simulink model "CanBusRagnar2020b"  (R2020b)
settings: Solver=VariableStepAuto  StartTime=0.0  StopTime=5.0  RelTol=1e-3
values from neighbouring files (symbols this model uses):
  F_mimo = -place(A,B,Desired_poles)    [SS_MIMO.m]    (also in controller_code.m = [ -230.9401         0         0         0  -34.4133         )
  sys_mimo = ss(A,B,C,0)    [SS_MIMO.m]
libraries: truetime x6, simulink_extras x4, dspsrcs4 x1
settings Model: Creator=mozzr  LastModifiedBy=krist
settings DebuggingCC: SFMachineParentedDataDiag=error

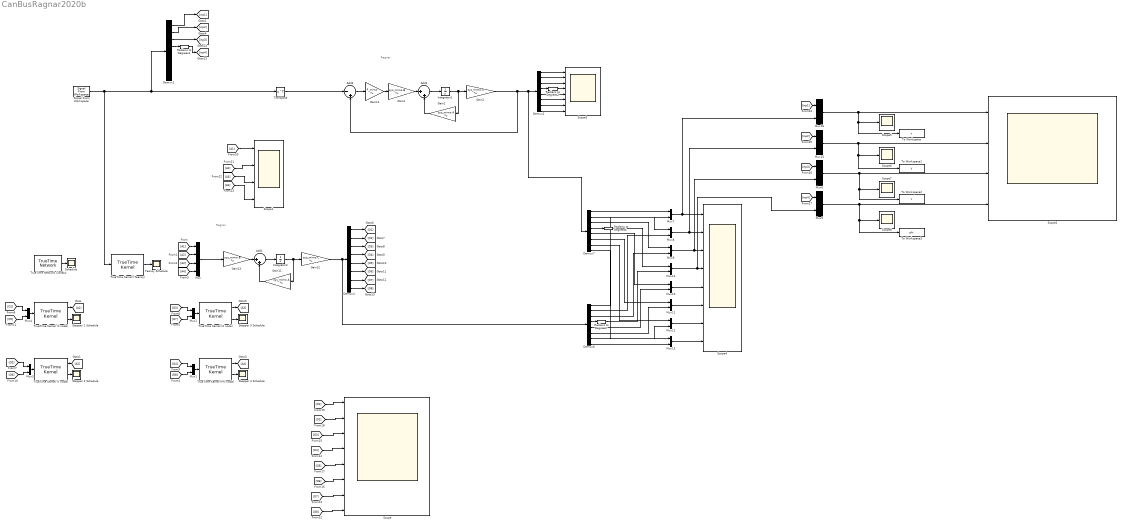
== system CanBusRagnar2020b ==
  note: Ragnar
  note: Ragnar
  Add1 : Sum  Inputs=|++
  Add2 : Sum  Inputs=|++
  Add3 : Sum  Inputs=|-+
  Demux{1..2,4,6..7} (5 alike) : Demux  Outputs=8
  Gain1 : Gain  Gain=sys_mimo.A  Multiplication=Matrix(K*u)
  Gain11 : Gain  Gain=sys_mimo.A  Multiplication=Matrix(K*u)
  Gain12 : Gain  Gain=sys_mimo.C  Multiplication=Matrix(K*u)
  Gain13 : Gain  Gain=sys_mimo.B  Multiplication=Matrix(K*u)
  Gain14 : Gain  Gain=F_mimo  Multiplication=Matrix(K*u)
  Gain2 : Gain  Gain=sys_mimo.C  Multiplication=Matrix(K*u)
  Gain3 : Gain  Gain=sys_mimo.B  Multiplication=Matrix(K*u)
  Integrator1 : Integrator  InitialCondition=[0 0.5 -0.4 deg2rad(90) 0 0 0 0]'
  Integrator2 : Integrator  InitialCondition=[0 0.5 -0.4 deg2rad(90) 0 0 0 0]
  Mux : Mux
  Mux{1..16} (16 alike) : Mux  Inputs=2
  Radians to Degrees{1..2,6..7} (4 alike) : simulink_extras/Transformations/Radians to Degrees
  Schedule : Scope
  Scope : Scope  NumInputPorts=8
  Scope1 : Scope  NumInputPorts=4
  Scope2 : Scope  NumInputPorts=4
  Scope3 : Scope  NumInputPorts=8
  Scope4 : Scope  NumInputPorts=8
  Scope{5..8} (4 alike) : Scope
  Signal From Workspace : dspsrcs4/Signal From Workspace  X=ref  Ts=1  nsamps=1  OutputAfterFinalValue=Holding final value  ignoreOrWarnInputAndFrameLengths=off  OutputFrames=off
  Stepper 1 Schedule : Scope
  Stepper 2 Schedule : Scope
  Stepper 3 Schedule : Scope
  Stepper 4 Schedule : Scope
  Teensy Schedule : Scope
  To Workspace : ToWorkspace  VariableName=x  SaveFormat=Timeseries  SampleTime=-1
  To Workspace1 : ToWorkspace  VariableName=y  SaveFormat=Timeseries  SampleTime=-1
  To Workspace2 : ToWorkspace  VariableName=z  SaveFormat=Timeseries  SampleTime=-1
  To Workspace3 : ToWorkspace  VariableName=phi  SaveFormat=Timeseries  SampleTime=-1
  Transpose : Math  Operator=transpose  SaturateOnIntegerOverflow=on
  TrueTime Kernel (Phi node) : truetime/TrueTime Kernel  sfun=nodePhi_init  args=[]  ninputsoutputs=[2 1]  ntriggers=0  trigtype=falling  nwnodenbr=[1 5]  clockoffsetdrift=[0 0]  schedoutput=on  battery=off  poweroutput=off  label=1: 5
  TrueTime Kernel (Teensy) : truetime/TrueTime Kernel  sfun=Teensy_init  args=[]  ninputsoutputs=[8 0]  ntriggers=0  trigtype=falling  nwnodenbr=[1 1]  clockoffsetdrift=[0 0]  schedoutput=on  battery=off  poweroutput=off  label=1: 1
  TrueTime Kernel (X node) : truetime/TrueTime Kernel  sfun=nodeX_init  args=[]  ninputsoutputs=[2 1]  ntriggers=0  trigtype=falling  nwnodenbr=[1 2]  clockoffsetdrift=[0 0]  schedoutput=on  battery=off  poweroutput=off  label=1: 2
  TrueTime Kernel (Y node) : truetime/TrueTime Kernel  sfun=nodeY_init  args=[]  ninputsoutputs=[2 1]  ntriggers=0  trigtype=falling  nwnodenbr=[1 3]  clockoffsetdrift=[0 0]  schedoutput=on  battery=off  poweroutput=off  label=1: 3
  TrueTime Kernel (Z node) : truetime/TrueTime Kernel  sfun=nodeZ_init  args=[]  ninputsoutputs=[2 1]  ntriggers=0  trigtype=falling  nwnodenbr=[1 4]  clockoffsetdrift=[0 0]  schedoutput=on  battery=off  poweroutput=off  label=1: 4
  TrueTime Network CanBus : truetime/TrueTime Network  nwtype=CSMA/AMP (CAN)  nwnbr=1  nnodes=5  rate=10000000  minsize=512  lossprob=0  seed=0  bandwidths=[0.5 0.5]  slotsize=512  schedule=[1 1 2]  memsize=80000  buftype=Common buffer  overflow=Retransmit  dynSchedule=0  miniSlotSize=0  NIT=0  QSortMode=FIFO  sync=0  irtSchedule=0  nrtLength=0  nodeGraph=0  scheduleoutput=on
  wires:
  TrueTime Kernel (Y node)/2 -> Stepper 2 Schedule/1
  TrueTime Kernel (X node)/2 -> Stepper 1 Schedule/1
  TrueTime Kernel (Phi node)/2 -> Stepper 4 Schedule/1
  TrueTime Kernel (Z node)/2 -> Stepper 3 Schedule/1
  TrueTime Kernel (Teensy)/1 -> Teensy Schedule/1
  TrueTime Network CanBus/1 -> Schedule/1
  TrueTime Kernel (X node)/1 -> [A1]
  [A1] -> Mux/1
  TrueTime Kernel (Y node)/1 -> [A2]
  TrueTime Kernel (Phi node)/1 -> [A4]
  TrueTime Kernel (Z node)/1 -> [A3]
  [A2] -> Mux/2
  [A3] -> Mux/3
  [A4] -> Mux/4
  Demux4/1 -> [O1]
  Demux4/2 -> [O2]
  Demux4/3 -> [O3]
  Demux4/4 -> [O4]
  Demux4/5 -> [O5]
  Demux4/6 -> [O6]
  Demux4/7 -> [O7]
  Demux4/8 -> [O8]
  Mux1/1 -> TrueTime Kernel (Phi node)/1
  [O4] -> Mux1/1
  [O8] -> Mux1/2
  [O3] -> Mux2/1
  [O7] -> Mux2/2
  Mux2/1 -> TrueTime Kernel (Z node)/1
  [O2] -> Mux3/1
  [O6] -> Mux3/2
  Mux3/1 -> TrueTime Kernel (Y node)/1
  [O1] -> Mux4/1
  [O5] -> Mux4/2
  Mux4/1 -> TrueTime Kernel (X node)/1
  Gain11/1 -> Add1/2
  Gain13/1 -> Add1/1
  Add1/1 -> Integrator2/1
  Mux/1 -> Gain13/1
  Integrator2/1 -> Gain11/1, Gain12/1
  [O8] -> Scope/8
  [O7] -> Scope/7
  [O4] -> Scope/4
  [O3] -> Scope/3
  [O5] -> Scope/5
  [O6] -> Scope/6
  [O2] -> Scope/2
  [O1] -> Scope/1
  [A1] -> Scope1/1
  [A2] -> Scope1/2
  [A3] -> Scope1/3
  [A4] -> Scope1/4
  Radians to Degrees2/1 -> Scope3/4
  Gain14/1 -> Gain3/1
  Add3/1 -> Gain14/1
  Integrator1/1 -> Gain1/1, Gain2/1
  Demux2/3 -> Scope3/3
  Demux2/2 -> Scope3/2
  Demux2/5 -> Scope3/5
  Demux2/8 -> Scope3/8
  Gain1/1 -> Add2/2
  Demux2/1 -> Scope3/1
  Add2/1 -> Integrator1/1
  Gain3/1 -> Add2/1
  Demux2/6 -> Scope3/6
  Demux2/7 -> Scope3/7
  Demux2/4 -> Radians to Degrees2/1
  Mux12/1 -> Scope4/7
  Mux7/1 -> Scope4/1, Mux16/2
  Demux6/5 -> Mux10/2
  Mux11/1 -> Scope4/6
  Demux7/7 -> Mux12/1
  Demux6/1 -> Mux7/2
  Radians to Degrees7/1 -> Mux14/2
  Demux6/6 -> Mux11/2
  Demux6/7 -> Mux12/2
  Demux7/2 -> Mux8/1
  Mux10/1 -> Scope4/5
  Demux6/2 -> Mux8/2
  Demux7/5 -> Mux10/1
  Mux13/1 -> Scope4/8
  Demux7/6 -> Mux11/1
  Radians to Degrees6/1 -> Mux14/1
  Demux6/8 -> Mux13/2
  Demux7/8 -> Mux13/1
  Mux14/1 -> Mux5/2, Scope4/4
  Gain2/1 -> Add3/2, Demux7/1, Demux2/1
  Demux6/4 -> Radians to Degrees7/1
  Demux6/3 -> Mux9/2
  Demux7/1 -> Mux7/1
  Mux9/1 -> Mux6/2, Scope4/3
  Gain12/1 -> Demux6/1, Demux4/1
  Demux7/4 -> Radians to Degrees6/1
  Demux7/3 -> Mux9/1
  Mux8/1 -> Mux15/2, Scope4/2
  Signal From Workspace/1 -> Demux1/1, Transpose/1, TrueTime Kernel (Teensy)/1
  Transpose/1 -> Add3/1
  Mux5/1 -> To Workspace3/1, Scope8/1, Scope2/4
  Mux6/1 -> To Workspace2/1, Scope7/1, Scope2/3
  Mux15/1 -> To Workspace1/1, Scope6/1, Scope2/2
  Mux16/1 -> To Workspace/1, Scope5/1, Scope2/1
  Demux1/4 -> Radians to Degrees1/1
  Demux1/1 -> [inp1]
  Demux1/2 -> [inp2]
  Demux1/3 -> [inp3]
  Radians to Degrees1/1 -> [inp4]
  [inp1] -> Mux16/1
  [inp2] -> Mux15/1
  [inp3] -> Mux6/1
  [inp4] -> Mux5/1
